simulink model "controlador_PID_DISCRETO"  (R2023b)
settings: Solver=VariableStepAuto  StartTime=0.0  StopTime=10.0  RelTol=1e-3
values from neighbouring files (symbols this model uses):
  b_a = J_eq*(2*zitta+1)*w_pos    (= 0.0395694444444)    [constantes.m]
  K_sa = J_eq*(2*zitta+1)*w_pos^2    (= 31.6555555556)    [constantes.m]    (also in test_polos_PID.m = J_eq*n*w_pos^2)
  K_sia = J_eq*w_pos^3    (= 10129.7777778)    [constantes.m]    (also in test_polos_PID.m = J_eq*w_pos^3)
  Ts = 2*pi/(10*5000)    (= 0.000125663706144)    [constantes.m]    (also in test_polos_PID.m = 40)
undefined symbols (not defined in the file or in its folder): DiscIntNeverNeededParam
settings Model: Creator=rodri  LastModifiedBy=Nahuel

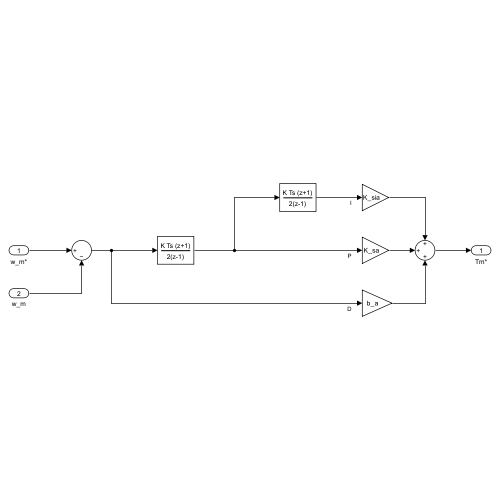
[thumbnail: Simulink's stored preview of the top-level diagram]
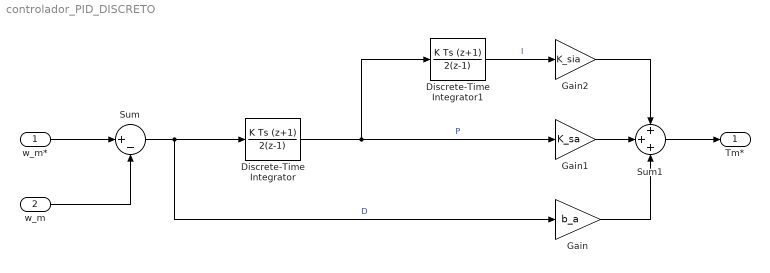
== system controlador_PID_DISCRETO ==
  w_m* : Inport
  w_m : Inport  Port=2
  Discrete-Time Integrator : DiscreteIntegrator  IntegratorMethod=Integration: Trapezoidal  SampleTime=Ts  ICPrevOutput=DiscIntNeverNeededParam  ICPrevScaledInput=DiscIntNeverNeededParam
  Discrete-Time Integrator1 : DiscreteIntegrator  IntegratorMethod=Integration: Trapezoidal  SampleTime=Ts  ICPrevOutput=DiscIntNeverNeededParam  ICPrevScaledInput=DiscIntNeverNeededParam
  Gain : Gain  Gain=b_a
  Gain1 : Gain  Gain=K_sa
  Gain2 : Gain  Gain=K_sia
  Sum : Sum  Inputs=|+-
  Sum1 : Sum  Inputs=+++
  Tm* : Outport
  wires:
  w_m*/1 -> Sum/1
  w_m/1 -> Sum/2
  Sum/1 -> Discrete-Time Integrator/1, Gain/1  "D"
  Gain2/1 -> Sum1/1
  Gain1/1 -> Sum1/2
  Gain/1 -> Sum1/3
  Sum1/1 -> Tm*/1
  Discrete-Time Integrator/1 -> Discrete-Time Integrator1/1, Gain1/1  "P"
  Discrete-Time Integrator1/1 -> Gain2/1  "I"
